simulink model "phase_loop_cosim"  (Simulink 7.8)
settings: Solver=ode23  StartTime=0.0  StopTime=1  RelTol=1e-3
model workspace (MAT data in the model file):
  DigitalFreq : Simulink.Parameter (value not decoded)
undefined symbols (not defined in the file or in its folder): a, b, DiscIntNeverNeededParam
libraries: simulink x12, modelsimlib x1
Description:
  | Complex Simulink model for PROPER phase_loop entity cosimulation
  | 
  | Correctly samples and filter input signal:
  | - Configure sampling process on the "Sampler" block
  | 
  | Generates all clocks and signals for the simulated block following a run/done interface:
  | - Configure digital clk generation on this model workspace
  |   * Change DigitalFreq model workspace variable
  | - run, rst and clk signals are generated using the model block
  | 
  | Correctly sets sampling frequencies for all signals.
  | 
  | Generates, on Matlab workspace, once simulation is finished or stopd, 2 variables:
  | 1) phase_loop_cosim_in
  |     Vector with the INPUT values to the phase_loop
  |     Each row is a SAMPLE.
  |     Has 4 columns:
  |     <initial columns> -> output values (check model)
  |     before last -> output sample time
  |        That is, this is not the simulation time of the input sample which resulted in this output value (a value which would be a little earlier in time).
  |        This is the EXACT time at which the done signal went up and the output was sapmled
  |     last -> Sample 3 (corresponding input sample #)
  | 2) phase_loop_cosim_out
  |     Format is identical to phase_loop_cosim_in vector, but this time sampled values are the input block values
  | 
  | === Usage ===
  | 1) Launch Modelsim from Matlab for Simulink cosimulation
  |     >> vsim('socketsimulink', 4449)
  | 2) Open the 'phase_loop' project, for easy compilation of spll design phase loop
  |      Location: spll/modelsim/phase_loop.mpf
  | 3) Compile project inside ModelSim
  | 4) Launch simulation using special simulation command for connecting VSIM with Matlab
  |     ModelSim> vsimulink work.phase_loop
settings Model: Creator=obmun  LastModifiedBy=obmun  SimulationMode=accelerator
settings OptimizationCC: SimCompilerOptimization=On

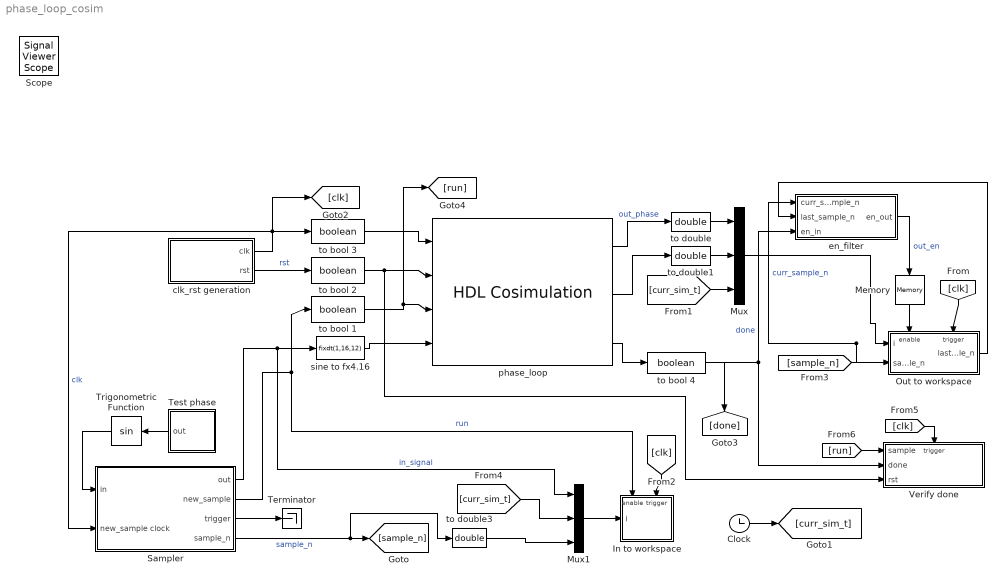
== system phase_loop_cosim ==
  Clock : Clock
  In to workspace : Subsystem  TreatAsAtomicUnit=on
  Memory : Memory  InheritSampleTime=on
  Mux : Mux  Inputs=3
  Mux1 : Mux  Inputs=3
  Out to workspace : Subsystem  TreatAsAtomicUnit=on
  Sampler : Subsystem  mask{f_s=1e4}
      mask prompts: f_s "Sample frequency (Hz"
      mask help:
      | The "sampler" block is a LPF + S&H entity, a helper block for connecting
      | Simulink continuous signals to a VHDL block following the 'run_done' inter-
      | face specs.
      |
      | It takes care of antialias-filtering an input signal and sampling it, as
      | well of generating the 'run' or 'sample' signal for the VHDL block.
      |
      | Sampling freq. can be setup using the equivalente block parameter. Internal
      | LPF antialias freq is automatically adjusted.
      |
      | An internal counter with current sample_n is maintained (starts at 0), and
      | sample_n is available as an output.
      |
      | ==== Input ports ====
      | == in ==
      | The values to be sampled. Can be a vector.
      |
      | == new_sample clock ==
      | Connect here the _digital_ clock used for driving the VHDL block. It's
      | required for correctly generating a just 1 cycle 'run' pulse for requesting
      | the begging of a new calculation to the connected 'run_done' interface.
      |
      | ==== Output ports ====
      | == out ==
      | The antialiased and held input vector
      |
      | == new_sample ==
      | This is the output for the 'run' signal generated by this block each time a
      | new sample is available.
      |
      | Each time a _new sample_ is available, a pulse of no more than 1 cycle of
      | 'new_sample clock' is generated.
      |
      | This pulse is generated the next rising edge after the new sample from 'in'
      |  signal has been taken, and it's delayed 1/4 of the new_sample clock. The
      | reason for this delay is to avoid problems inside the VHDL simulation when
      | the input signals rise at the _same_ exact time as the clock signal (which
      | we know it's not a sane way of doing things in the _real_ digital IC world).
      |
      | == trigger ==
      | This is a COPY of the internal trigger signal used to sample input value.
      |
      | == sample_n ==
      | Signal with the CURRENT sample number. The output of the internal sample counter. Type: integer.
      |
      | That is, before anything has been sampled, the output of this port is -1.
      | AFTER 1 sample is being hold, the ouput is 0, and so on.
      mask init:
      | [b, a] = sampler_block_init(gcb, f_s);
  Terminator : Terminator
  Test phase : Subsystem
      mask init:
      | phase_jump_selector = [0 0;...
      | 2.4*(1/50) 1;...
      | (2.4 + 2.8)*(1/50) 2;...
      | (2.4 + 2.8 + 3)*(1/50) 3];
      | freq_jump_selector = [0 0;...
      |      3*(1/50) 1;...
      |      3*(1/50) + 3*(1/51) 2];
  Trigonometric Function : Trigonometry
  Verify done : Subsystem  Description=|  TreatAsAtomicUnit=on
      | This block takes care of verifying that the 'done' signal of the run_done interface ALWAYS is rised by the block veying analized before a new SAMPLE is ready.
      |                                                                                                                                                               
      | That means that what we're checking here is that the iterative block under verification is FAST ENOUGH to keep with the input values rate
  clk_rst generation : Subsystem  mask{clk_f=DigitalFreq}
      mask prompts: clk_f "Clock frequency (Hz)"
      mask help:
      | Este bloque se encarga de generar una señal de reloj de frecuencia indicada
      | por el usuario mediante el parámetro correspondiente.
      | La salida reloj comienza en valor 0 y sube a 1 tras 1/2 del período espe-
      | cificado, generando el primer flanco ascendente.
      |
      | Desde el comienzo de la simulación hasta poco después de este primer flanco
      |  ascendente, mantiene la salida 'rst' a 1 para permitir situar en un esta-
      | do controlado aquellos bloques secuenciales que la señal de reloj controle.
      mask init:
      | rst_signal = [0, 1; 3/(4*clk_f), 0];
  en_filter : Subsystem
  phase_loop : modelsimlib/HDL Cosimulation  PortPaths=/phase_loop/clk;/phase_loop/rst;/phase_loop/run;/phase_loop/norm_input;/phase_loop/phase;/phase_loop/norm_sin;/phase_loop/done  PortModes=[1 1 1 1 2 2 2 ]  PortTimes=[-1,-1,-1,-1,1/(2*DigitalFreq),1/(2*DigitalFreq),1/(2*DigitalFreq)]  PortSigns=[-1 -1 -1 -1 1 1 -1 ]  PortFracLengths=[0,0,0,0,12,12,0]  CommLocal=on  CommSharedMemory=on  CommPortNumber=4449  CommShowInfo=on  ClockModes=[]  ClockTimes=[]  TclPreSimCommand="puts \"Running Simulink Cosimulation block.\""  TclPostSimCommand="puts \"done\""  TimingMode=s  TimingScaleFactor=1  idxCellArray={'UNUSED_VAR'}  CosimBypass=Full Simulation  AllowDirectFeedthrough=off  ProductName=EDA Simulator Link MQ  RunAutoTimescale=off  HdlClocks=0
  sine to fx4.16 : DataTypeConversion  OutDataTypeStr=fixdt(1,16,12)  RndMeth=Nearest  SaturateOnIntegerOverflow=on
  to bool {1..4} (4 alike) : DataTypeConversion  OutDataTypeStr=boolean  RndMeth=Nearest  SaturateOnIntegerOverflow=on
  to double : DataTypeConversion  OutDataTypeStr=double
  to double1 : DataTypeConversion  OutDataTypeStr=double
  to double3 : DataTypeConversion  OutDataTypeStr=double
  Scope : SignalViewerScope  IOType=viewer  NumInputPorts=6  ZoomMode=xonly  RefreshTime=0.035000
      settings: TickLabels=on  TimeRange=0.00012  YMin=0~-5~-1~-1~0~0  YMax=1~5~8~8~1~1
  wires:
  Sampler/1(out) -> sine to fx4.16/1, Mux1/1  "in_signal"
  Sampler/2(new_sample) -> to bool 1/1, In to workspace/Enable  "run"
  clk_rst generation/1(clk) -> Sampler/2(new_sample clock), [clk], to bool 3/1  "clk"
  clk_rst generation/2(rst) -> to bool 2/1  "rst"
  Trigonometric Function/1 -> Sampler/1(in)
  to bool 2/1 -> Verify done/3(rst), phase_loop/2
  to bool 1/1 -> [run], phase_loop/3
  to bool 4/1 -> Verify done/2(done), [done], en_filter/3(en_in)  "done"
  phase_loop/1 -> to double/1  "out_phase"
  Sampler/3(trigger) -> Terminator/1
  Test phase/1(out) -> Trigonometric Function/1
  Sampler/4(sample_n) -> to double3/1, [sample_n]  "sample_n"
  Clock/1 -> [curr_sim_t]
  Mux/1 -> Out to workspace/1(i)
  [clk] -> Out to workspace/Trigger
  [clk] -> In to workspace/Trigger
  Mux1/1 -> In to workspace/1(i)
  to double/1 -> Mux/1
  to double1/1 -> Mux/2
  [sample_n] -> en_filter/1(curr_sample_n), Out to workspace/2(sample_n)  "curr_sample_n"
  [curr_sim_t] -> Mux/3
  [clk] -> Verify done/Trigger
  en_filter/1(en_out) -> Memory/1  "out_en"
  Out to workspace/1(last_sample_n) -> en_filter/2(last_sample_n)
  Memory/1 -> Out to workspace/Enable
  [run] -> Verify done/1(sample)
  phase_loop/2 -> to double1/1
  phase_loop/3 -> to bool 4/1
  to bool 3/1 -> phase_loop/1
  sine to fx4.16/1 -> phase_loop/4
  [curr_sim_t] -> Mux1/2
  to double3/1 -> Mux1/3

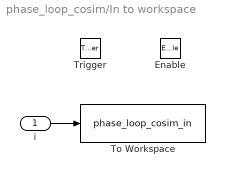
== system phase_loop_cosim/In to workspace ==
  i : Inport
  Enable : EnablePort
  Trigger : TriggerPort
  To Workspace : ToWorkspace  VariableName=phase_loop_cosim_in  SampleTime=-1  SaveFormat=Array
  wires:
  i/1 -> To Workspace/1

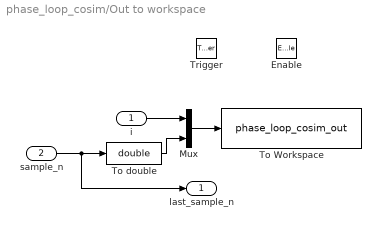
== system phase_loop_cosim/Out to workspace ==
  i : Inport
  sample_n : Inport  Port=2
  Enable : EnablePort
  Trigger : TriggerPort
  Mux : Mux  Inputs=2
  To Workspace : ToWorkspace  VariableName=phase_loop_cosim_out  SampleTime=-1  SaveFormat=Array
  To double : DataTypeConversion  OutDataTypeStr=double
  last_sample_n : Outport  InitialOutput=-1
  wires:
  i/1 -> Mux/1
  Mux/1 -> To Workspace/1
  To double/1 -> Mux/2
  sample_n/1 -> To double/1, last_sample_n/1

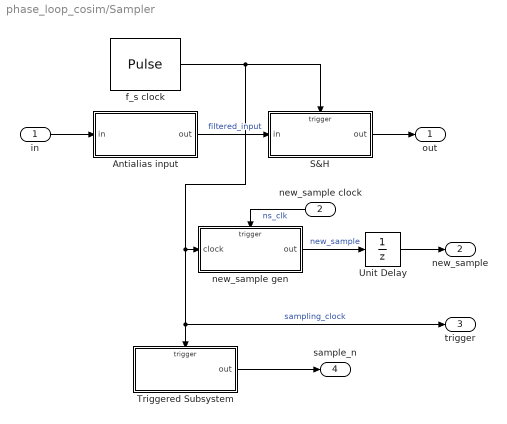
== system phase_loop_cosim/Sampler ==
  in : Inport
  new_sample clock : Inport  Port=2
  Antialias input : Subsystem  TreatAsAtomicUnit=on
  S&H : Subsystem  TreatAsAtomicUnit=on
  Triggered Subsystem : Subsystem  TreatAsAtomicUnit=on
  Unit Delay : UnitDelay  Description=|  SampleTime=-1
      | Esta ruta posee un sample rate dado por la señal de reloj (new_sample_clock).                                                                                                                                                                                                                                                                            
      |                                                                                                                                                                                                                                                                                                                                                          
      | Analicemos que valor tendrá aquí el "retardo unitario". Teniendo en cuenta la forma de generar el reloj digital de entrada por 'new_sample clock' que tenemos, el sampling rate en este bloque es de un sample cada 1/4 de período de señal de reloj de entrada por 'new_sample clock', es decir, la señal de reloj para los bloques cosimulados de VHDL.
      |                                                                                                                                                                                                                                                                                                                                                          
      | Por lo tanto, el retardo unitario será 1/4 de período del reloj digital externo.                                                                                                                                                                                                                                                                         
      |                                                                                                                                                                                                                                                                                                                                                          
      | La idea de introducir este retardo es para _evitar_ que la señal 'new_sample' suba y baje en el mismo instante de tiempo que el reloj digital al bloque VHDL. Así, al retrasarlo un 1/4 de ciclo de reloj, el bloque detectará la orden de 'sample' en el siguiente ciclo de reloj                                                                       
      |                                                                                                                                                                                                                                                                                                                                                          
      | De manera efectiva, este bloque retarda 1/4 de período de reloj la señal de sample.                                                                                                                                                                                                                                                                      
      |                                                                                                                                                                                                                                                                                                                                                          
      | El motivo: de lo contrario el SAMPLE sube a '1' _justo_ en el flanco ascendente de reloj de la PLL, y no nos interesan estasn coincidencias tan sutiles (recordemos las deltas en VHDL). Para que el sistema digital la coja, conviene retardarlo para que la orden de 'sample' sea enganchada en el siguiente ciclo de reloj digital
  f_s clock : DiscretePulseGenerator  Period=4  PulseWidth=2  PhaseDelay=1  SampleTime=1/(4*f_s)
  new_sample gen : Subsystem  TreatAsAtomicUnit=on
  out : Outport
  new_sample : Outport  Port=2
  trigger : Outport  Port=3
  sample_n : Outport  Port=4
  wires:
  in/1 -> Antialias input/1(in)
  S&H/1(out) -> out/1
  Antialias input/1(out) -> S&H/1(in)  "filtered_input"
  new_sample gen/1(out) -> Unit Delay/1  "new_sample"
  f_s clock/1 -> S&H/Trigger, new_sample gen/1(clock), trigger/1, Triggered Subsystem/Trigger  "sampling_clock"
  new_sample clock/1 -> new_sample gen/Trigger  "ns_clk"
  Unit Delay/1 -> new_sample/1
  Triggered Subsystem/1(out) -> sample_n/1

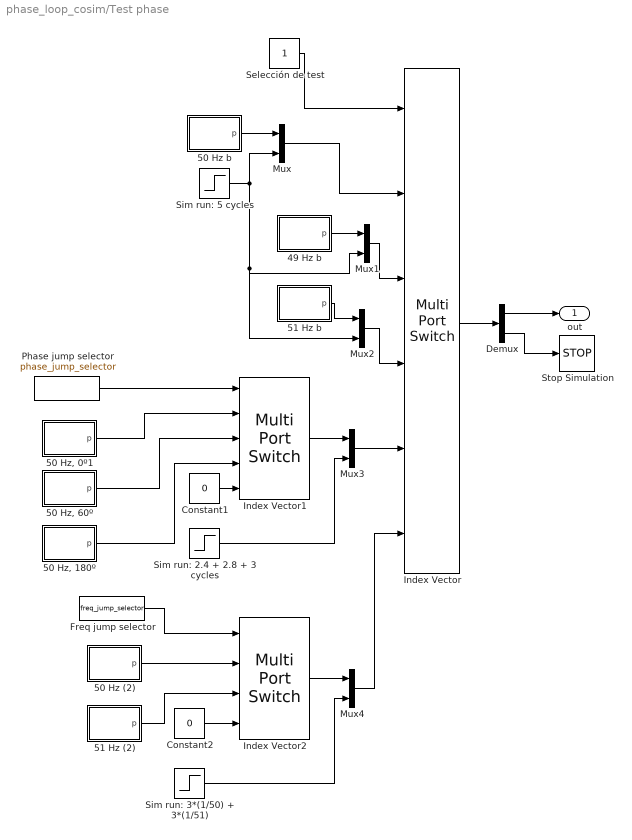
== system phase_loop_cosim/Test phase ==
  49 Hz b : Subsystem
  50 Hz (2) : Subsystem
  50 Hz b : Subsystem
  "50 Hz, 0º1" : Subsystem
  "50 Hz, 180º" : Subsystem
  "50 Hz, 60º" : Subsystem
  51 Hz (2) : Subsystem
  51 Hz b : Subsystem
  Constant1 : Constant  Value=0
  Constant2 : Constant  Value=0
  Demux : Demux  Outputs=2
  Freq jump selector : FromWorkspace  VariableName=freq_jump_selector  SampleTime=0  Interpolate=off  OutputAfterFinalValue=Holding final value
  Index Vector : MultiPortSwitch  DataPortOrder=Zero-based contiguous  Inputs=5  zeroidx=on
  Index Vector1 : MultiPortSwitch  DataPortOrder=Zero-based contiguous  Inputs=4  zeroidx=on
  Index Vector2 : MultiPortSwitch  DataPortOrder=Zero-based contiguous  zeroidx=on
  Mux{,1..4} (5 alike) : Mux  Inputs=2
  Phase jump selector : FromWorkspace  VariableName=phase_jump_selector  SampleTime=0  Interpolate=off  OutputAfterFinalValue=Holding final value
  Selección de test : Constant
  Sim run: 2.4 + 2.8 + 3 cycles : Step  Time=(2.4 + 2.8 + 3)*(1/50)  SampleTime=0
  Sim run: 3*(1/50) + 3*(1/51) : Step  Time=3*(1/50) + 3*(1/51)  SampleTime=0
  Sim run: 5 cycles : Step  Time=10*(1/50)  SampleTime=0
  Stop Simulation : Stop
  out : Outport
  wires:
  Selección de test/1 -> Index Vector/1
  Phase jump selector/1 -> Index Vector1/1
  Constant1/1 -> Index Vector1/5
  Constant2/1 -> Index Vector2/4
  Freq jump selector/1 -> Index Vector2/1
  "50 Hz, 0º1"/1(p) -> Index Vector1/2
  "50 Hz, 60º"/1(p) -> Index Vector1/3
  "50 Hz, 180º"/1(p) -> Index Vector1/4
  50 Hz (2)/1(p) -> Index Vector2/2
  51 Hz (2)/1(p) -> Index Vector2/3
  50 Hz b/1(p) -> Mux/1
  Sim run: 5 cycles/1 -> Mux/2, Mux1/2, Mux2/2
  Mux/1 -> Index Vector/2
  Index Vector/1 -> Demux/1
  Demux/1 -> out/1
  Demux/2 -> Stop Simulation/1
  49 Hz b/1(p) -> Mux1/1
  Mux1/1 -> Index Vector/3
  51 Hz b/1(p) -> Mux2/1
  Mux2/1 -> Index Vector/4
  Index Vector1/1 -> Mux3/1
  Mux3/1 -> Index Vector/5
  Sim run: 2.4 + 2.8 + 3 cycles/1 -> Mux3/2
  Index Vector2/1 -> Mux4/1
  Sim run: 3*(1/50) + 3*(1/51)/1 -> Mux4/2
  Mux4/1 -> Index Vector/6

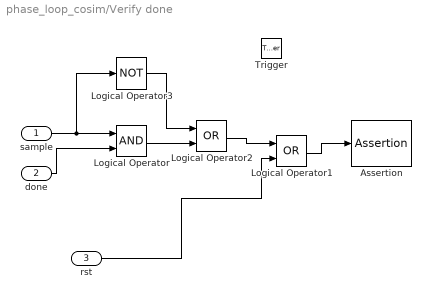
== system phase_loop_cosim/Verify done ==
  sample : Inport
  done : Inport  Port=2
  rst : Inport  Port=3
  Trigger : TriggerPort
  Assertion : Assertion  Enabled=on
  Logical Operator : Logic  AllPortsSameDT=off  OutDataTypeStr=boolean
  Logical Operator1 : Logic  Operator=OR  AllPortsSameDT=off  OutDataTypeStr=boolean
  Logical Operator2 : Logic  Operator=OR  AllPortsSameDT=off  OutDataTypeStr=boolean
  Logical Operator3 : Logic  Operator=NOT  AllPortsSameDT=off  OutDataTypeStr=boolean
  wires:
  sample/1 -> Logical Operator/1, Logical Operator3/1
  done/1 -> Logical Operator/2
  Logical Operator1/1 -> Assertion/1
  rst/1 -> Logical Operator1/2
  Logical Operator3/1 -> Logical Operator2/1
  Logical Operator/1 -> Logical Operator2/2
  Logical Operator2/1 -> Logical Operator1/1

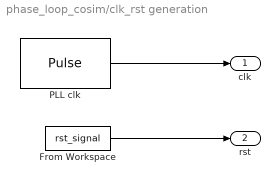
== system phase_loop_cosim/clk_rst generation ==
  From Workspace : FromWorkspace  VariableName=rst_signal  SampleTime=1/(4*clk_f)  Interpolate=off  OutputAfterFinalValue=Holding final value
  PLL clk : DiscretePulseGenerator  Period=4  PulseWidth=2  PhaseDelay=2  SampleTime=1/(4*clk_f)
  clk : Outport
  rst : Outport  Port=2
  wires:
  PLL clk/1 -> clk/1
  From Workspace/1 -> rst/1

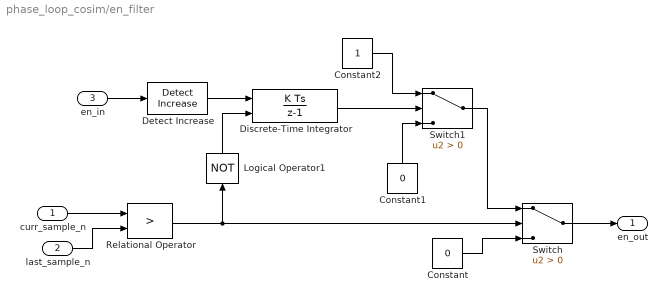
== system phase_loop_cosim/en_filter ==
  curr_sample_n : Inport
  last_sample_n : Inport  Port=2
  en_in : Inport  Port=3
  Constant : Constant  Value=0
  Constant1 : Constant  Value=0
  Constant2 : Constant
  Detect Increase : simulink/Logic and Bit Operations/Detect Increase  vinit=0.0  InputProcessing=Inherited  OutDataTypeStr=boolean
  Discrete-Time Integrator : DiscreteIntegrator  ExternalReset=level  SampleTime=-1  OutDataTypeStr=double  LimitOutput=on  UpperSaturationLimit=1  LowerSaturationLimit=0  ICPrevOutput=DiscIntNeverNeededParam  ICPrevScaledInput=DiscIntNeverNeededParam
  Logical Operator1 : Logic  Operator=NOT  AllPortsSameDT=off  OutDataTypeStr=boolean
  Relational Operator : RelationalOperator  Operator=>  OutDataTypeStr=boolean
  Switch : Switch  Criteria=u2 > Threshold
  Switch1 : Switch  Criteria=u2 > Threshold
  en_out : Outport
  wires:
  Relational Operator/1 -> Switch/2, Logical Operator1/1
  curr_sample_n/1 -> Relational Operator/1
  last_sample_n/1 -> Relational Operator/2
  Detect Increase/1 -> Discrete-Time Integrator/1
  en_in/1 -> Detect Increase/1
  Discrete-Time Integrator/1 -> Switch1/2
  Switch1/1 -> Switch/1
  Constant2/1 -> Switch1/1
  Constant1/1 -> Switch1/3
  Constant/1 -> Switch/3
  Switch/1 -> en_out/1
  Logical Operator1/1 -> Discrete-Time Integrator/2

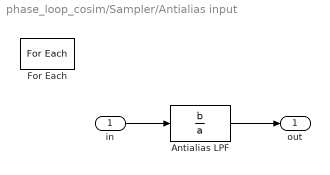
== system phase_loop_cosim/Sampler/Antialias input ==
  in : Inport  Partition=on  PartitionDimension=1  PartitionWidth=1
  Antialias LPF : TransferFcn  Numerator=b  Denominator=a
  For Each : ForEach  DisableCoverage=on  IndexMode=One-based
  out : Outport  ConcatenationDimension=1
  wires:
  in/1 -> Antialias LPF/1
  Antialias LPF/1 -> out/1

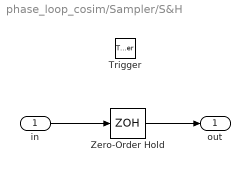
== system phase_loop_cosim/Sampler/S&H ==
  in : Inport
  Trigger : TriggerPort
  Zero-Order Hold : ZeroOrderHold  SampleTime=-1
  out : Outport
  wires:
  in/1 -> Zero-Order Hold/1
  Zero-Order Hold/1 -> out/1

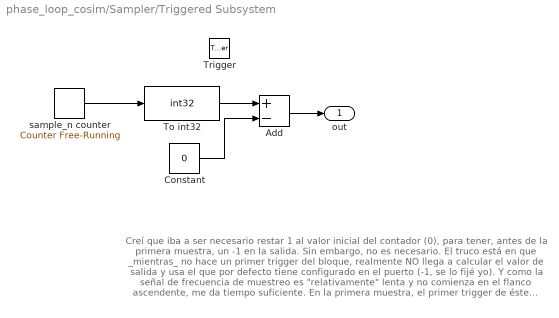
== system phase_loop_cosim/Sampler/Triggered Subsystem ==
  note: Creí que iba a ser necesario restar 1 al valor inicial del contador (0), para tener, antes de la primera muestra, un -1 en la salida.
      | Sin embargo, no es necesario.
      | El truco está en que _mientras_ no hace un primer trigger del bloque, realmente NO llega a calcular el valor de salida y usa el que
      | por defecto tiene configurado en el puerto (-1, se lo fijé yo).
      | Y como la señal de frecuencia de muestreo es "relativamente" lenta y no comienza en el flanco ascendente, me da tiempo suficiente.
      |
      | En la primera muestra, el primer trigger de éste bloque y otros muchos, es el primer flanco ascendente, que lo que hace es inicializar el counter.
      | Entonces, en lugar de sacar 1, es la primera inicialización y sale un 0.
  Trigger : TriggerPort
  Add : Sum  Inputs=+-
  Constant : Constant  Value=0  OutDataTypeStr=int32
  To int32 : DataTypeConversion  OutDataTypeStr=int32
  sample_n counter : simulink/Sources/Counter Free-Running  NumBits=31  tsamp=-1
  out : Outport  InitialOutput=-1
  wires:
  sample_n counter/1 -> To int32/1
  To int32/1 -> Add/1
  Add/1 -> out/1
  Constant/1 -> Add/2

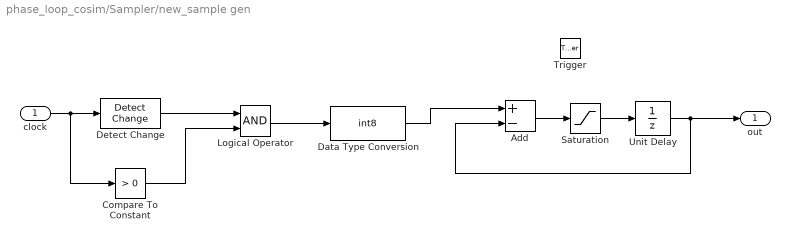
== system phase_loop_cosim/Sampler/new_sample gen ==
  clock : Inport
  Trigger : TriggerPort
  Add : Sum  Inputs=+-
  Compare To Constant : simulink/Logic and Bit Operations/Compare To Constant  relop=>  const=0  OutDataTypeStr=boolean
  Data Type Conversion : DataTypeConversion  OutDataTypeStr=int8
  Detect Change : simulink/Logic and Bit Operations/Detect Change  vinit=0  InputProcessing=Inherited  OutDataTypeStr=boolean
  Logical Operator : Logic  AllPortsSameDT=off  OutDataTypeStr=boolean
  Saturation : Saturate  UpperLimit=1  LowerLimit=0
  Unit Delay : UnitDelay  SampleTime=-1
  out : Outport  InitialOutput=0
  wires:
  clock/1 -> Detect Change/1, Compare To Constant/1
  Unit Delay/1 -> Add/2, out/1
  Detect Change/1 -> Logical Operator/1
  Logical Operator/1 -> Data Type Conversion/1
  Data Type Conversion/1 -> Add/1
  Add/1 -> Saturation/1
  Saturation/1 -> Unit Delay/1
  Compare To Constant/1 -> Logical Operator/2

== system phase_loop_cosim/Test phase/49 Hz b ==
  49 Hz ramp : simulink/Sources/Ramp  slope=2*pi*49  start=0  X0=0
  mod 2pi : MATLABFcn  MATLABFcn=mod(u, 2*pi)
  p : Outport
  wires:
  49 Hz ramp/1 -> mod 2pi/1
  mod 2pi/1 -> p/1

== system phase_loop_cosim/Test phase/50 Hz (2) ==
  50 Hz ramp : simulink/Sources/Ramp  slope=2*pi*50  start=0  X0=0
  mod 2pi : MATLABFcn  MATLABFcn=mod(u, 2*pi)
  p : Outport
  wires:
  50 Hz ramp/1 -> mod 2pi/1
  mod 2pi/1 -> p/1

== system phase_loop_cosim/Test phase/50 Hz b ==
  50 Hz ramp : simulink/Sources/Ramp  slope=2*pi*50  start=0  X0=0
  mod 2pi : MATLABFcn  MATLABFcn=mod(u, 2*pi)
  p : Outport
  wires:
  50 Hz ramp/1 -> mod 2pi/1
  mod 2pi/1 -> p/1

== system phase_loop_cosim/Test phase/50 Hz, 0º1 ==
  50 Hz ramp : simulink/Sources/Ramp  slope=2*pi*50  start=0  X0=0
  mod 2pi : MATLABFcn  MATLABFcn=mod(u, 2*pi)
  p : Outport
  wires:
  50 Hz ramp/1 -> mod 2pi/1
  mod 2pi/1 -> p/1

== system phase_loop_cosim/Test phase/50 Hz, 180º ==
  "50 Hz, 180º ramp" : simulink/Sources/Ramp  slope=2*pi*50  start=0  X0=(180/180)*pi
  mod 2pi : MATLABFcn  MATLABFcn=mod(u, 2*pi)
  p : Outport
  wires:
  "50 Hz, 180º ramp"/1 -> mod 2pi/1
  mod 2pi/1 -> p/1

== system phase_loop_cosim/Test phase/50 Hz, 60º ==
  "50 Hz, 60º ramp" : simulink/Sources/Ramp  slope=2*pi*50  start=0  X0=(60/180)*pi
  mod 2pi : MATLABFcn  MATLABFcn=mod(u, 2*pi)
  p : Outport
  wires:
  "50 Hz, 60º ramp"/1 -> mod 2pi/1
  mod 2pi/1 -> p/1

== system phase_loop_cosim/Test phase/51 Hz (2) ==
  51 Hz ramp : simulink/Sources/Ramp  slope=2*pi*51  start=0  X0=0
  mod 2pi : MATLABFcn  MATLABFcn=mod(u, 2*pi)
  p : Outport
  wires:
  51 Hz ramp/1 -> mod 2pi/1
  mod 2pi/1 -> p/1

== system phase_loop_cosim/Test phase/51 Hz b ==
  51 Hz ramp : simulink/Sources/Ramp  slope=2*pi*51  start=0  X0=0
  mod 2pi : MATLABFcn  MATLABFcn=mod(u, 2*pi)
  p : Outport
  wires:
  51 Hz ramp/1 -> mod 2pi/1
  mod 2pi/1 -> p/1
